simulink model "untitled1"  (R2023a)
settings: Solver=VariableStepAuto  StartTime=0.0  StopTime=10.0  RelTol=1e-3
model workspace (MAT data in the model file):
  L = 1
  X = Simulink.Parameter
  X.DataType = '<data type expression>'
  X.Complexity = 'real'
  X.Dimensions = [0 0]
  g = 9.81
values from neighbouring files (symbols this model uses):
  B = [b11 ... (first row only)    [bicyclekinematicmodel.m]    (also in constants.m = 10; newbike.m = 0; newbikemodel.m = 0; newnewbike.m = 10)
  C = [1,0;0,1]    [bicyclekinematicmodel.m]    (also in constants.m = 0.0002787; newbike.m = 0; newbikemodel.m = 0; newnewbike.m = 0.0002787)
  J = (pi/2) * (r^4)    (= 0.0186284035067)    [constants.m]    (also in newnewbike.m)
  lambda = 0.05    [constants.m]    (also in newnewbike.m)
  m = 12    [bicyclekinematicmodel.m]    (also in constants.m = 1000; newbike.m; newbikemodel.m; newnewbike.m = 1000)
  r = 0.33    [constants.m]    (also in newnewbike.m)
  theta0 = theta    (= 1.57079632679)    [newnewbike.m]
settings Model: Creator=smath24  LastModifiedBy=smath24

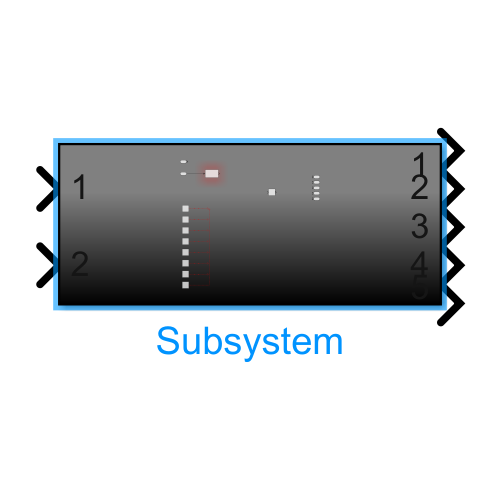
[thumbnail: Simulink's stored preview of the top-level diagram]
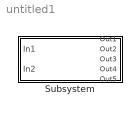
== system untitled1 ==
  Subsystem : Subsystem

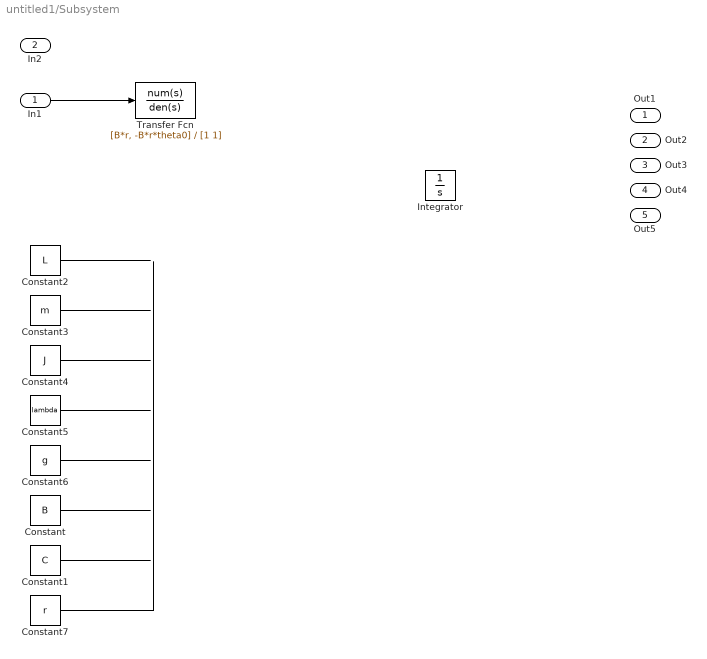
== system untitled1/Subsystem ==
  In1 : Inport
  In2 : Inport  Port=2
  Constant : Constant  Value=B
  Constant1 : Constant  Value=C
  Constant2 : Constant  Value=L
  Constant3 : Constant  Value=m
  Constant4 : Constant  Value=J
  Constant5 : Constant  Value=lambda
  Constant6 : Constant  Value=g
  Constant7 : Constant  Value=r
  Integrator : Integrator
  Transfer Fcn : TransferFcn  Numerator=[B*r, -B*r*theta0]  Denominator=[1 1]
  Out1 : Outport
  Out2 : Outport  Port=2
  Out3 : Outport  Port=3
  Out4 : Outport  Port=4
  Out5 : Outport  Port=5
  wires:
  In1/1 -> Transfer Fcn/1
  Constant6/1 -> ?
  Constant2/1 -> ?
  Constant/1 -> ?
  Constant5/1 -> ?
  Constant3/1 -> ?
  Constant1/1 -> ?
  Constant4/1 -> ?
  Constant7/1 -> ?
